simulink model "Three_Phase_AC_Voltage_Controller"  (R2021b)
settings: Solver=ode23tb  StartTime=0.0  StopTime=0.1  MaxStep=1e-4  RelTol=1e-3
undefined symbols (not defined in the file): k, m, n
libraries: spsThyristorLib x18, spsACVoltageSourceLib x9, spsCurrentMeasurementLib x9, spsSeriesRLCBranchLib x9, spsRMSLib x3, spsVoltageMeasurementLib x3, spspowerguiLib x1
settings Model: Creator=90542  LastModifiedBy=90542

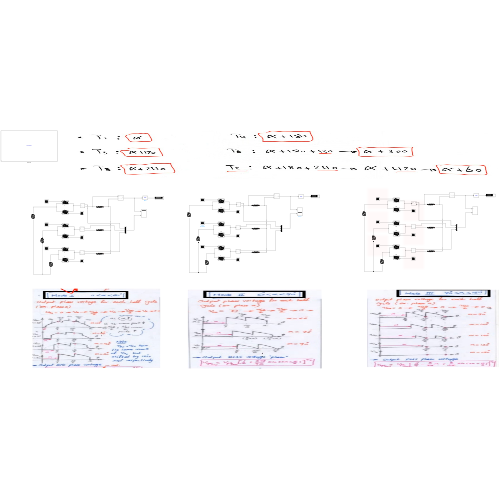
[thumbnail: Simulink's stored preview of the top-level diagram]
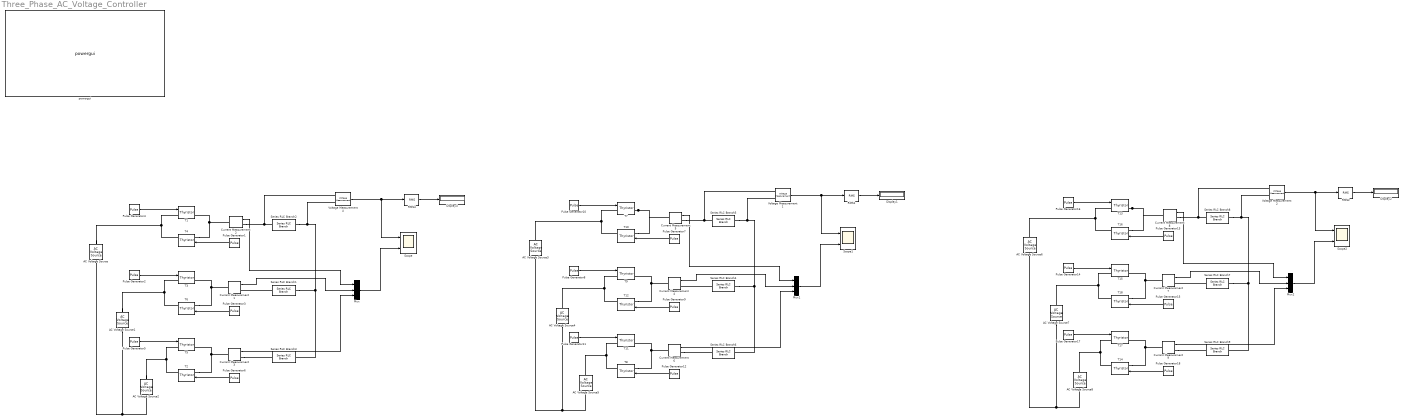
== system Three_Phase_AC_Voltage_Controller ==
  AC Voltage Source : spsACVoltageSourceLib/AC Voltage Source  Amplitude=100  Phase=0  Frequency=50  SampleTime=0  Measurements=None  BusType=swing  Pref=10e3  Qref=0  Qmin=-inf  Qmax=+inf
  AC Voltage Source1 : spsACVoltageSourceLib/AC Voltage Source  Amplitude=100  Phase=-120  Frequency=50  SampleTime=0  Measurements=None  BusType=swing  Pref=10e3  Qref=0  Qmin=-inf  Qmax=+inf
  AC Voltage Source2 : spsACVoltageSourceLib/AC Voltage Source  Amplitude=100  Phase=120  Frequency=50  SampleTime=0  Measurements=None  BusType=swing  Pref=10e3  Qref=0  Qmin=-inf  Qmax=+inf
  AC Voltage Source3 : spsACVoltageSourceLib/AC Voltage Source  Amplitude=100  Phase=0  Frequency=50  SampleTime=0  Measurements=None  BusType=swing  Pref=10e3  Qref=0  Qmin=-inf  Qmax=+inf
  AC Voltage Source4 : spsACVoltageSourceLib/AC Voltage Source  Amplitude=100  Phase=-120  Frequency=50  SampleTime=0  Measurements=None  BusType=swing  Pref=10e3  Qref=0  Qmin=-inf  Qmax=+inf
  AC Voltage Source5 : spsACVoltageSourceLib/AC Voltage Source  Amplitude=100  Phase=120  Frequency=50  SampleTime=0  Measurements=None  BusType=swing  Pref=10e3  Qref=0  Qmin=-inf  Qmax=+inf
  AC Voltage Source6 : spsACVoltageSourceLib/AC Voltage Source  Amplitude=100  Phase=0  Frequency=50  SampleTime=0  Measurements=None  BusType=swing  Pref=10e3  Qref=0  Qmin=-inf  Qmax=+inf
  AC Voltage Source7 : spsACVoltageSourceLib/AC Voltage Source  Amplitude=100  Phase=-120  Frequency=50  SampleTime=0  Measurements=None  BusType=swing  Pref=10e3  Qref=0  Qmin=-inf  Qmax=+inf
  AC Voltage Source8 : spsACVoltageSourceLib/AC Voltage Source  Amplitude=100  Phase=120  Frequency=50  SampleTime=0  Measurements=None  BusType=swing  Pref=10e3  Qref=0  Qmin=-inf  Qmax=+inf
  Current Measurement{1..9} (9 alike) : spsCurrentMeasurementLib/Current Measurement  PhasorSimulation=off  OutputType=Complex  PSBequivalent=0
  Display1 : Display
  Display2 : Display
  Display4 : Display
  Mux : Mux  Inputs=3
  Mux1 : Mux  Inputs=3
  Mux2 : Mux  Inputs=3
  Pulse Generator1 : DiscretePulseGenerator  PulseType=Time based  Amplitude=5  Period=0.02  PulseWidth=60  PhaseDelay=(k+180)*(0.02/360)
  Pulse Generator10 : DiscretePulseGenerator  PulseType=Time based  Amplitude=5  Period=0.02  PulseWidth=60  PhaseDelay=m*(0.02/360)
  Pulse Generator11 : DiscretePulseGenerator  PulseType=Time based  Amplitude=5  Period=0.02  PulseWidth=60  PhaseDelay=(m+240)*(0.02/360)
  Pulse Generator12 : DiscretePulseGenerator  PulseType=Time based  Amplitude=5  Period=0.02  PulseWidth=60  PhaseDelay=(m+60)*(0.02/360)
  Pulse Generator13 : DiscretePulseGenerator  PulseType=Time based  Amplitude=5  Period=0.02  PulseWidth=60  PhaseDelay=(n+180)*(0.02/360)
  Pulse Generator14 : DiscretePulseGenerator  PulseType=Time based  Amplitude=5  Period=0.02  PulseWidth=60  PhaseDelay=(n+120)*(0.02/360)
  Pulse Generator15 : DiscretePulseGenerator  PulseType=Time based  Amplitude=5  Period=0.02  PulseWidth=60  PhaseDelay=(n+300)*(0.02/360)
  Pulse Generator16 : DiscretePulseGenerator  PulseType=Time based  Amplitude=5  Period=0.02  PulseWidth=60  PhaseDelay=n*(0.02/360)
  Pulse Generator17 : DiscretePulseGenerator  PulseType=Time based  Amplitude=5  Period=0.02  PulseWidth=60  PhaseDelay=(n+240)*(0.02/360)
  Pulse Generator18 : DiscretePulseGenerator  PulseType=Time based  Amplitude=5  Period=0.02  PulseWidth=60  PhaseDelay=(n+60)*(0.02/360)
  Pulse Generator2 : DiscretePulseGenerator  PulseType=Time based  Amplitude=5  Period=0.02  PulseWidth=60  PhaseDelay=(k+120)*(0.02/360)
  Pulse Generator3 : DiscretePulseGenerator  PulseType=Time based  Amplitude=5  Period=0.02  PulseWidth=60  PhaseDelay=(k+300)*(0.02/360)
  Pulse Generator4 : DiscretePulseGenerator  PulseType=Time based  Amplitude=5  Period=0.02  PulseWidth=60  PhaseDelay=k*(0.02/360)
  Pulse Generator5 : DiscretePulseGenerator  PulseType=Time based  Amplitude=5  Period=0.02  PulseWidth=60  PhaseDelay=(k+240)*(0.02/360)
  Pulse Generator6 : DiscretePulseGenerator  PulseType=Time based  Amplitude=5  Period=0.02  PulseWidth=60  PhaseDelay=(k+60)*(0.02/360)
  Pulse Generator7 : DiscretePulseGenerator  PulseType=Time based  Amplitude=5  Period=0.02  PulseWidth=60  PhaseDelay=(m+180)*(0.02/360)
  Pulse Generator8 : DiscretePulseGenerator  PulseType=Time based  Amplitude=5  Period=0.02  PulseWidth=60  PhaseDelay=(m+120)*(0.02/360)
  Pulse Generator9 : DiscretePulseGenerator  PulseType=Time based  Amplitude=5  Period=0.02  PulseWidth=60  PhaseDelay=(m+300)*(0.02/360)
  RMS1 : spsRMSLib/RMS  TrueRMS=on  Freq=60  RMSInit=120  Ts=0
  RMS2 : spsRMSLib/RMS  TrueRMS=on  Freq=60  RMSInit=120  Ts=0
  RMS4 : spsRMSLib/RMS  TrueRMS=on  Freq=60  RMSInit=120  Ts=0
  Scope : Scope  NumInputPorts=2
  Scope1 : Scope  NumInputPorts=2
  Scope2 : Scope  NumInputPorts=2
  Series RLC Branch{1..9} (9 alike) : spsSeriesRLCBranchLib/Series RLC Branch  LConnTagsString=__new0  RConnTagsString=__new0  BranchType=R  Resistance=10  Inductance=20e-3  SetiL0=off  InitialCurrent=0  Capacitance=1e-6  Setx0=off  InitialVoltage=0  Measurements=None
  T{1..18} (18 alike) : spsThyristorLib/Thyristor  Ron=0.001  Lon=0  Vf=0.8  IC=0  Rs=500  Cs=250e-9  Measurements=on
  Voltage Measurement1 : spsVoltageMeasurementLib/Voltage Measurement  PhasorSimulation=off  OutputType=Complex  PSBequivalent=0
  Voltage Measurement2 : spsVoltageMeasurementLib/Voltage Measurement  PhasorSimulation=off  OutputType=Complex  PSBequivalent=0
  Voltage Measurement4 : spsVoltageMeasurementLib/Voltage Measurement  PhasorSimulation=off  OutputType=Complex  PSBequivalent=0
  powergui : spspowerguiLib/powergui  Priority=1  SimulationMode=Continuous  SampleTime=50e-6  frequency=60  Iterations=50  frequencyindice=50  Pbase=100e6  ErrMax=1e-4  UnitsV=kV  UnitsW=MW  buscounter=0  FunctionMessages=off  echomessages=off  EnableUseOfTLC=off  CurrentSourceSwitches=off  DisableSnubberDevices=off  DisableRonSwitches=off  DisableVfSwitches=off  DisplayEquations=off  AutomaticDiscreteSolvers=off  SolverType=Tustin/Backward Euler (TBE)  Interpol=off  ExternalGateDelay=off  methode=off  Ts=100  x0status=blocks  SPID=on  SwTol=0  HookPort=off  NonlinearTolerance=1e-4  nMaxIteration=100  ContinueOnMaxIteration=off  RestoreLinks=warning  ResistiveCurrentMeasurement=off  Frange=[0:2:500]  Ylog=off  Xlog=on  ShowGrid=off  save=off  variable=ZData  structure=0  ZoomFFT=off  StartTime=0.0  cycles=1  DisplayStyle=1  fundamental=60  FreqAxis=off  MaxFrequency=1000  frequencyindicesteady=1  RmsSteady=1  display=off
  wires:
  Pulse Generator4/1 -> T1/1
  Pulse Generator1/1 -> T4/1
  Pulse Generator3/1 -> T6/1
  Pulse Generator2/1 -> T3/1
  Pulse Generator5/1 -> T5/1
  Pulse Generator6/1 -> T2/1
  Current Measurement1/1 -> Mux/2
  Current Measurement2/1 -> Mux/1
  Current Measurement3/1 -> Mux/3
  Voltage Measurement4/1 -> RMS4/1, Scope/1
  Mux/1 -> Scope/2
  RMS4/1 -> Display4/1
  Pulse Generator11/1 -> T11/1
  Pulse Generator12/1 -> T8/1
  Pulse Generator7/1 -> T10/1
  Pulse Generator8/1 -> T9/1
  Current Measurement4/1 -> Mux1/2
  Mux1/1 -> Scope1/2
  Current Measurement5/1 -> Mux1/1
  Voltage Measurement1/1 -> RMS1/1, Scope1/1
  Pulse Generator10/1 -> T7/1
  RMS1/1 -> Display1/1
  Current Measurement6/1 -> Mux1/3
  Pulse Generator9/1 -> T12/1
  Pulse Generator17/1 -> T17/1
  Pulse Generator18/1 -> T14/1
  Pulse Generator13/1 -> T16/1
  Pulse Generator14/1 -> T15/1
  Current Measurement7/1 -> Mux2/2
  Mux2/1 -> Scope2/2
  Current Measurement8/1 -> Mux2/1
  Voltage Measurement2/1 -> RMS2/1, Scope2/1
  Pulse Generator16/1 -> T13/1
  RMS2/1 -> Display2/1
  Current Measurement9/1 -> Mux2/3
  Pulse Generator15/1 -> T18/1
  connections:
  T4/RConn1 -- AC Voltage Source/RConn1 -- T1/LConn1
  T4/LConn1 -- Current Measurement2/LConn1 -- T1/RConn1
  T6/LConn1 -- Current Measurement1/LConn1 -- T3/RConn1
  T6/RConn1 -- AC Voltage Source1/RConn1 -- T3/LConn1
  T2/LConn1 -- Current Measurement3/LConn1 -- T5/RConn1
  T2/RConn1 -- AC Voltage Source2/RConn1 -- T5/LConn1
  Current Measurement2/RConn1 -- Voltage Measurement4/LConn1 -- Series RLC Branch2/RConn1
  Series RLC Branch1/RConn1 -- Current Measurement1/RConn1
  Current Measurement3/RConn1 -- Series RLC Branch3/RConn1
  Series RLC Branch2/LConn1 -- Series RLC Branch1/LConn1 -- Series RLC Branch3/LConn1 -- Voltage Measurement4/LConn2
  AC Voltage Source1/LConn1 -- AC Voltage Source2/LConn1 -- AC Voltage Source/LConn1
  T8/RConn1 -- AC Voltage Source5/RConn1 -- T11/LConn1
  Series RLC Branch5/LConn1 -- Series RLC Branch4/LConn1 -- Series RLC Branch6/LConn1 -- Voltage Measurement1/LConn2
  T12/RConn1 -- AC Voltage Source4/RConn1 -- T9/LConn1
  T7/RConn1 -- T10/LConn1 -- Current Measurement5/LConn1
  AC Voltage Source4/LConn1 -- AC Voltage Source5/LConn1 -- AC Voltage Source3/LConn1
  T12/LConn1 -- Current Measurement4/LConn1 -- T9/RConn1
  Current Measurement5/RConn1 -- Voltage Measurement1/LConn1 -- Series RLC Branch5/RConn1
  T10/RConn1 -- AC Voltage Source3/RConn1 -- T7/LConn1
  T8/LConn1 -- Current Measurement6/LConn1 -- T11/RConn1
  Series RLC Branch4/RConn1 -- Current Measurement4/RConn1
  Current Measurement6/RConn1 -- Series RLC Branch6/RConn1
  T14/RConn1 -- AC Voltage Source8/RConn1 -- T17/LConn1
  Series RLC Branch8/LConn1 -- Series RLC Branch7/LConn1 -- Series RLC Branch9/LConn1 -- Voltage Measurement2/LConn2
  T18/RConn1 -- AC Voltage Source7/RConn1 -- T15/LConn1
  T13/RConn1 -- T16/LConn1 -- Current Measurement8/LConn1
  AC Voltage Source7/LConn1 -- AC Voltage Source8/LConn1 -- AC Voltage Source6/LConn1
  T18/LConn1 -- Current Measurement7/LConn1 -- T15/RConn1
  Current Measurement8/RConn1 -- Voltage Measurement2/LConn1 -- Series RLC Branch8/RConn1
  T16/RConn1 -- AC Voltage Source6/RConn1 -- T13/LConn1
  T14/LConn1 -- Current Measurement9/LConn1 -- T17/RConn1
  Series RLC Branch7/RConn1 -- Current Measurement7/RConn1
  Current Measurement9/RConn1 -- Series RLC Branch9/RConn1
